simulink model "iio_sink_sim"  (R2014a)
settings: Solver=ode45  StartTime=0.0  StopTime=inf  RelTol=1e-3
settings Model: Creator=ACozma  LastModifiedBy=ACozma
settings DebuggingCC: UnderspecifiedInitializationDetection=Classic

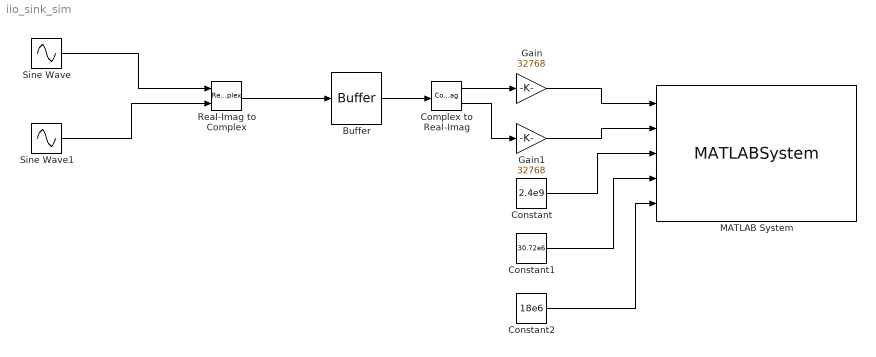
== system iio_sink_sim ==
  Buffer : Buffer  N=32768  TreatMby1Signals=One channel
  Complex to Real-Imag : ComplexToRealImag
  Constant : Constant  Value=2.4e9
  Constant1 : Constant  Value=30.72e6
  Constant2 : Constant  Value=18e6
  Gain : Gain  Gain=32768
  Gain1 : Gain  Gain=32768
  MATLAB System : MATLABSystem  System=iio_sys_obj_sink  SimulateUsing=Interpreted execution  ip_address=10.50.1.147  dev_name=ad9361  ch_size=32768  ch_no=2
      mask Type: iio_sys_obj_sink
      mask Display:
      | disp('ad9361 source');
      | port_label('input',1,'In1');
      | port_label('input',2,'In2');
      | port_label('input',3,'LO_FREQ');
      | port_label('input',4,'SAMPLING_FREQ');
      | port_label('input',5,'RF_BANDWIDTH');
  Real-Imag to Complex : RealImagToComplex
  Sine Wave : Sin  SineType=Sample based  Frequency=10  Samples=100  SampleTime=1
  Sine Wave1 : Sin  SineType=Sample based  Frequency=10  Phase=90  Samples=100  SampleTime=1  Offset=75
  wires:
  Complex to Real-Imag/1 -> Gain/1
  Complex to Real-Imag/2 -> Gain1/1
  Gain/1 -> MATLAB System/1
  Buffer/1 -> Complex to Real-Imag/1
  Sine Wave/1 -> Real-Imag to Complex/1
  Sine Wave1/1 -> Real-Imag to Complex/2
  Real-Imag to Complex/1 -> Buffer/1
  Gain1/1 -> MATLAB System/2
  Constant/1 -> MATLAB System/3
  Constant1/1 -> MATLAB System/4
  Constant2/1 -> MATLAB System/5
